simulink model "Buckfsattempt"  (R2022b)
settings: Solver=VariableStepAuto  StartTime=0.0  StopTime=2  RelTol=1e-3
values from neighbouring files (symbols this model uses):
  angular_corner_freq = ( (n^3*(1-D)^2*R_L + (n-D*(n-1)*r_l) ) / (L_m*C*(R_L + r_c)*(n-D*(n-1)) ) )^0.5    (= 137999.679282)    [Worspace.m]
  C_min = D/(R_L*fsw*Output_V_rip)    (= 9.6e-05)    [Worspace.m]
  D = 0.4    [Model_Worksapce.mat]    (also in Worspace.m = 0.5)
  damp_ratio = tau/(2*(rho*gamma)^0.5)    (= 0.148310872127)    [Worspace.m]
  fsw = 100000    [Model_Worksapce.mat]    (also in Worspace.m)
  Gain_Constant = ( (n^2*D*D_n*R_L*r_c ) / (L_m*(R_L + r_c)*(n-D*(n-1))) )    (= 22245.3945082)    [Worspace.m]
  L_m = 0.25    [Model_Worksapce.mat]    (also in Worspace.m = 3.41796875e-07)
  N1 = 24    [Model_Worksapce.mat]    (also in Worspace.m)
  N2 = 72    [Model_Worksapce.mat]    (also in Worspace.m = 48)
  N2_N1 = 3    [Model_Worksapce.mat]    (also in Worspace.m = 2)
  P_out = 50    [Model_Worksapce.mat]    (also in Worspace.m)
  R_L = 1.04166666667    [Model_Worksapce.mat]    (also in Worspace.m)
  Vs = 24    [Model_Worksapce.mat]    (also in Worspace.m)
  w_zn = 1/(C*r_c)    (= 104166.666667)    [Worspace.m]
libraries: spsCurrentMeasurementLib x10, spsSeriesRLCBranchLib x10, spsVoltageMeasurementLib x7, spsDCVoltageSourceLib x5, spsControlledCurrentSourceLib x2, spsControlledVoltageSourceLib x2, spsDiodeLib x2, spsIdealSwitchLib x2, spsMeanLib x2, spsPWMGeneratorDCDCLib x2, spsParallelRLCBranchLib x1, spsLinearTransformerLib x1
settings Model: Creator=enese  LastModifiedBy=enese

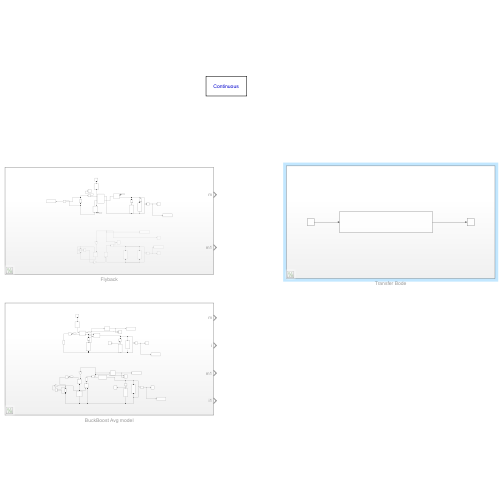
[thumbnail: Simulink's stored preview of the top-level diagram]
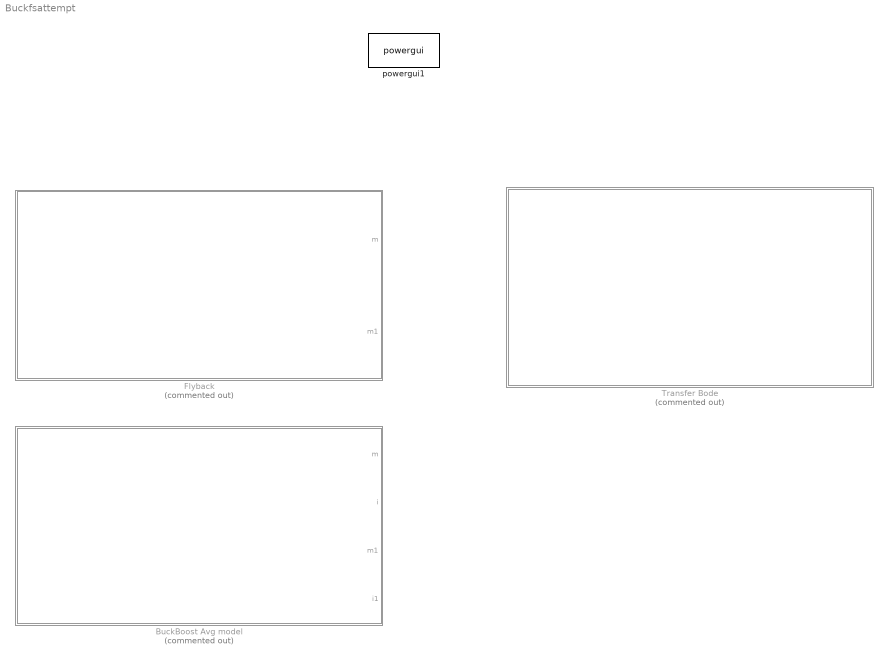
== system Buckfsattempt ==
  BuckBoost Avg model : Subsystem  Commented=on
  Flyback : Subsystem  Commented=on
  Transfer Bode : Subsystem  Commented=on
  powergui1 : spspowerguiLib/powergui  Priority=1  SimulationMode=Continuous  SampleTime=50e-6  frequency=60  Iterations=50  frequencyindice=0  Pbase=100e6  ErrMax=1e-4  UnitsV=kV  UnitsW=MW  buscounter=0  FunctionMessages=off  echomessages=off  EnableUseOfTLC=off  CurrentSourceSwitches=off  DisableSnubberDevices=off  DisableRonSwitches=off  DisableVfSwitches=off  DisplayEquations=off  AutomaticDiscreteSolvers=off  SolverType=Tustin/Backward Euler (TBE)  Interpol=off  ExternalGateDelay=off  methode=off  Ts=100  x0status=blocks  SPID=on  SwTol=0  HookPort=off  NonlinearTolerance=1e-4  nMaxIteration=100  ContinueOnMaxIteration=off  RestoreLinks=warning  ResistiveCurrentMeasurement=off  Frange=[0:2:500]  Ylog=off  Xlog=on  ShowGrid=off  save=off  variable=ZData  structure=0  ZoomFFT=off  StartTime=0.0  cycles=1  DisplayStyle=1  fundamental=60  FreqAxis=off  MaxFrequency=1000  frequencyindicesteady=1  RmsSteady=1  display=off

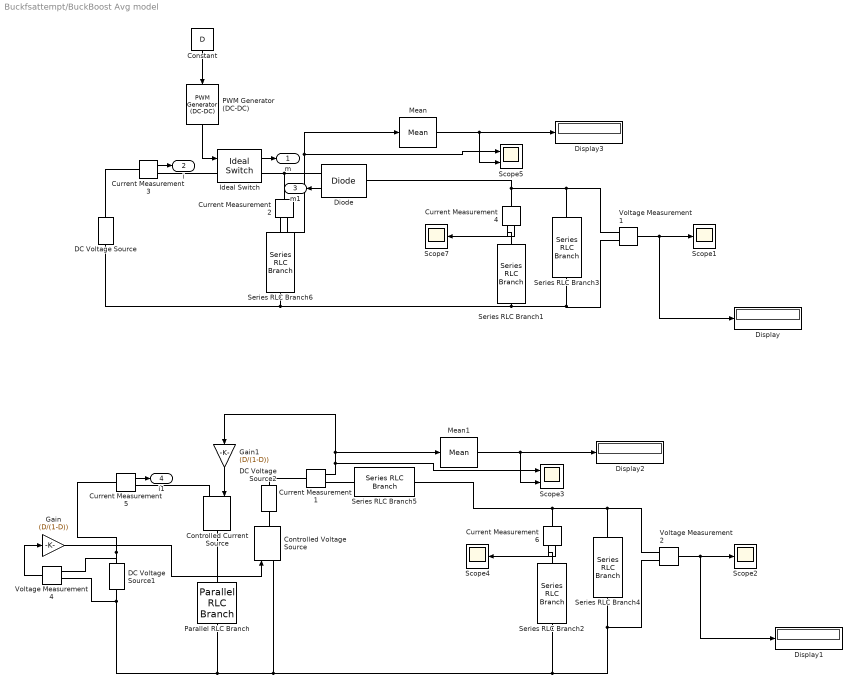
== system Buckfsattempt/BuckBoost Avg model ==
  Constant : Constant  Value=D
  Controlled Current Source : spsControlledCurrentSourceLib/Controlled Current Source  Initialize=on  Source_Type=DC  Amplitude=0  Phase=0  Frequency=0  Measurements=None
  Controlled Voltage Source : spsControlledVoltageSourceLib/Controlled Voltage Source  Initialize=on  Source_Type=DC  Amplitude=0  Phase=0  Frequency=0  Measurements=None
  Current Measurement{1..6} (6 alike) : spsCurrentMeasurementLib/Current Measurement  PhasorSimulation=off  OutputType=Complex  PSBequivalent=0
  DC Voltage Source : spsDCVoltageSourceLib/DC Voltage Source  Amplitude=Vs  Measurements=Voltage
  DC Voltage Source1 : spsDCVoltageSourceLib/DC Voltage Source  Amplitude=Vs  Measurements=Voltage
  DC Voltage Source2 : spsDCVoltageSourceLib/DC Voltage Source  Amplitude=0  Measurements=Voltage
  Diode : spsDiodeLib/Diode  Ron=0.001  Lon=0  Vf=0.8  IC=0  UseSnubber=0  Rs=500  Cs=250e-9  Measurements=on
  Display{,1..3} (4 alike) : Display
  Gain : Gain  Gain=(D/(1-D))
  Gain1 : Gain  Gain=(D/(1-D))
  Ideal Switch : spsIdealSwitchLib/Ideal Switch  Ron=0.001  Lon=0  IC=0  Rs=1e5  Cs=inf  Measurements=on
  Mean : spsMeanLib/Mean  Freq=100e3  Vinit=0  Ts=0
  Mean1 : spsMeanLib/Mean  Freq=100e3  Vinit=0  Ts=0
  PWM Generator (DC-DC) : spsPWMGeneratorDCDCLib/PWM Generator (DC-DC)  Fsw=100e3  Ts=0
  Parallel RLC Branch : spsParallelRLCBranchLib/Parallel RLC Branch  LConnTagsString=a  RConnTagsString=__new0  BranchType=RL  Resistance=1e10  Inductance=20e-6  SetiL0=off  InitialCurrent=0  Capacitance=1e-6  Setx0=off  InitialVoltage=0  Measurements=None
  Scope{1..2,4,7} (4 alike) : Scope
  Scope3 : Scope  NumInputPorts=2
  Scope5 : Scope  NumInputPorts=2
  Series RLC Branch1 : spsSeriesRLCBranchLib/Series RLC Branch  LConnTagsString=__new0  RConnTagsString=__new0  BranchType=C  Resistance=50e-7  Inductance=1e-3  SetiL0=off  InitialCurrent=0  Capacitance=80e-6  Setx0=off  InitialVoltage=0  Measurements=None
  Series RLC Branch2 : spsSeriesRLCBranchLib/Series RLC Branch  LConnTagsString=__new0  RConnTagsString=__new0  BranchType=C  Resistance=50e-7  Inductance=1e-3  SetiL0=off  InitialCurrent=0  Capacitance=80e-6  Setx0=off  InitialVoltage=0  Measurements=None
  Series RLC Branch3 : spsSeriesRLCBranchLib/Series RLC Branch  LConnTagsString=__new0  RConnTagsString=__new0  BranchType=R  Resistance=5  Inductance=1e-3  SetiL0=off  InitialCurrent=0  Capacitance=20e-6  Setx0=off  InitialVoltage=0  Measurements=None
  Series RLC Branch4 : spsSeriesRLCBranchLib/Series RLC Branch  LConnTagsString=__new0  RConnTagsString=__new0  BranchType=R  Resistance=5  Inductance=1e-3  SetiL0=off  InitialCurrent=0  Capacitance=20e-6  Setx0=off  InitialVoltage=0  Measurements=None
  Series RLC Branch5 : spsSeriesRLCBranchLib/Series RLC Branch  LConnTagsString=__new0  RConnTagsString=__new0  BranchType=L  Resistance=50e-7  Inductance=1e-3  SetiL0=off  InitialCurrent=0  Capacitance=80e-6  Setx0=off  InitialVoltage=0  Measurements=None
  Series RLC Branch6 : spsSeriesRLCBranchLib/Series RLC Branch  LConnTagsString=__new0  RConnTagsString=__new0  BranchType=L  Resistance=50e-7  Inductance=20e-6  SetiL0=off  InitialCurrent=0  Capacitance=470e-6  Setx0=off  InitialVoltage=0  Measurements=None
  Voltage Measurement1 : spsVoltageMeasurementLib/Voltage Measurement  PhasorSimulation=off  OutputType=Complex  PSBequivalent=0
  Voltage Measurement2 : spsVoltageMeasurementLib/Voltage Measurement  PhasorSimulation=off  OutputType=Complex  PSBequivalent=0
  Voltage Measurement4 : spsVoltageMeasurementLib/Voltage Measurement  PhasorSimulation=off  OutputType=Complex  PSBequivalent=0
  m : Outport
  i : Outport  Port=2
  m1 : Outport  Port=3
  i1 : Outport  Port=4
  wires:
  Gain/1 -> Controlled Voltage Source/1
  PWM Generator (DC-DC)/1 -> Ideal Switch/1
  Mean1/1 -> Display2/1, Scope3/2
  Voltage Measurement4/1 -> Gain/1
  Ideal Switch/1 -> m/1
  Voltage Measurement1/1 -> Scope1/1, Display/1
  Constant/1 -> PWM Generator (DC-DC)/1
  Current Measurement1/1 -> Scope3/1, Mean1/1, Gain1/1
  Voltage Measurement2/1 -> Display1/1, Scope2/1
  Gain1/1 -> Controlled Current Source/1
  Current Measurement4/1 -> Scope7/1
  Mean/1 -> Scope5/2, Display3/1
  Current Measurement2/1 -> Mean/1, Scope5/1
  Current Measurement6/1 -> Scope4/1
  Current Measurement3/1 -> i/1
  Diode/1 -> m1/1
  Current Measurement5/1 -> i1/1
  connections:
  Ideal Switch/RConn1 -- Current Measurement2/LConn1 -- Diode/RConn1
  Current Measurement6/RConn1 -- Series RLC Branch2/LConn1
  Voltage Measurement2/LConn2 -- Series RLC Branch4/RConn1 -- Series RLC Branch2/RConn1 -- Parallel RLC Branch/RConn1 -- Voltage Measurement4/LConn1 -- DC Voltage Source1/LConn1 -- Controlled Voltage Source/LConn1
  Voltage Measurement2/LConn1 -- Series RLC Branch4/LConn1 -- Series RLC Branch5/RConn1 -- Current Measurement6/LConn1
  Series RLC Branch3/RConn1 -- DC Voltage Source/LConn1 -- Series RLC Branch6/LConn1 -- Series RLC Branch1/RConn1 -- Voltage Measurement1/LConn2
  Current Measurement2/RConn1 -- Series RLC Branch6/RConn1
  Current Measurement1/LConn1 -- DC Voltage Source2/RConn1
  Series RLC Branch5/LConn1 -- Current Measurement1/RConn1
  Voltage Measurement1/LConn1 -- Diode/LConn1 -- Current Measurement4/LConn1 -- Series RLC Branch3/LConn1
  Current Measurement5/LConn1 -- Voltage Measurement4/LConn2 -- DC Voltage Source1/RConn1
  Current Measurement4/RConn1 -- Series RLC Branch1/LConn1
  Ideal Switch/LConn1 -- Current Measurement3/RConn1
  Controlled Current Source/LConn1 -- Current Measurement5/RConn1
  Current Measurement3/LConn1 -- DC Voltage Source/RConn1
  Parallel RLC Branch/LConn1 -- Controlled Current Source/RConn1
  DC Voltage Source2/LConn1 -- Controlled Voltage Source/RConn1

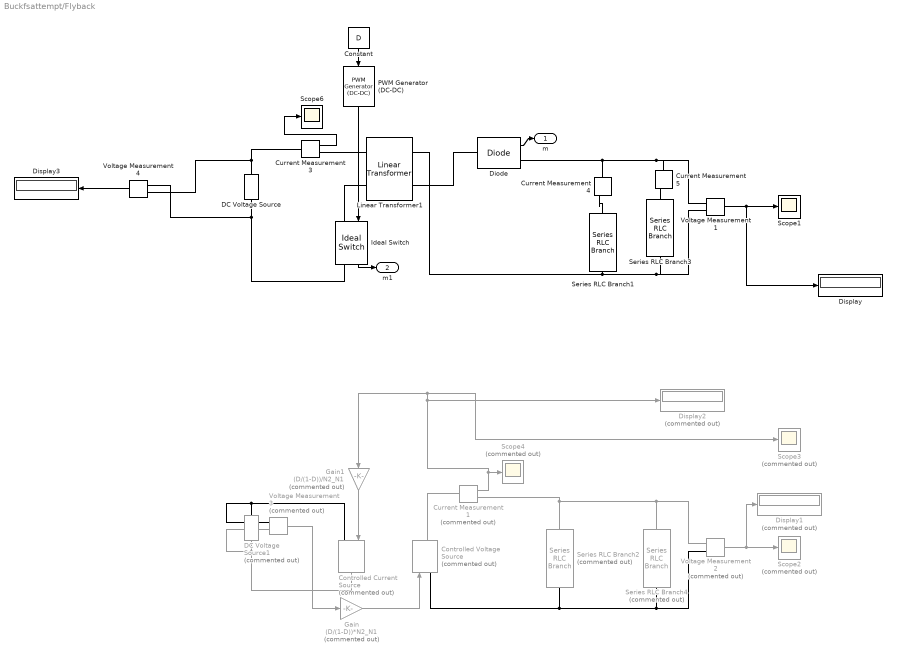
== system Buckfsattempt/Flyback ==
  Constant : Constant  Value=D
  Controlled Current Source : spsControlledCurrentSourceLib/Controlled Current Source  Commented=on  Initialize=on  Source_Type=DC  Amplitude=0  Phase=0  Frequency=0  Measurements=None
  Controlled Voltage Source : spsControlledVoltageSourceLib/Controlled Voltage Source  Commented=on  Initialize=on  Source_Type=DC  Amplitude=0  Phase=0  Frequency=0  Measurements=None
  Current Measurement1 : spsCurrentMeasurementLib/Current Measurement  Commented=on  PhasorSimulation=off  OutputType=Complex  PSBequivalent=0
  Current Measurement3 : spsCurrentMeasurementLib/Current Measurement  PhasorSimulation=off  OutputType=Complex  PSBequivalent=0
  Current Measurement4 : spsCurrentMeasurementLib/Current Measurement  PhasorSimulation=off  OutputType=Complex  PSBequivalent=0
  Current Measurement5 : spsCurrentMeasurementLib/Current Measurement  PhasorSimulation=off  OutputType=Complex  PSBequivalent=0
  DC Voltage Source : spsDCVoltageSourceLib/DC Voltage Source  Amplitude=Vs  Measurements=Voltage
  DC Voltage Source1 : spsDCVoltageSourceLib/DC Voltage Source  Commented=on  Amplitude=Vs  Measurements=Voltage
  Diode : spsDiodeLib/Diode  Ron=0.001  Lon=0  Vf=0.8  IC=0  UseSnubber=0  Rs=800  Cs=250e-9  Measurements=on
  Display : Display
  Display1 : Display  Commented=on
  Display2 : Display  Commented=on
  Display3 : Display
  Gain : Gain  Commented=on  Gain=(D/(1-D))*N2_N1
  Gain1 : Gain  Commented=on  Gain=(D/(1-D))/N2_N1
  Ideal Switch : spsIdealSwitchLib/Ideal Switch  Ron=0.001  Lon=0  IC=0  Rs=1e5  Cs=inf  Measurements=on
  Linear Transformer1 : spsLinearTransformerLib/Linear Transformer  UNITS=SI  NominalPower=[ P_out fsw ]  winding1=[N1 0 0]  winding2="[N2 0  0]"  ThreeWindings=off  winding3=[3.15e+05 3.969e+07 6316.9]  RmLm=[10e8 L_m*1.05]  Measurements=None  DataType=on
  PWM Generator (DC-DC) : spsPWMGeneratorDCDCLib/PWM Generator (DC-DC)  Fsw=fsw  Ts=0
  Scope1 : Scope
  Scope2 : Scope  Commented=on
  Scope3 : Scope  Commented=on
  Scope4 : Scope  Commented=on
  Scope6 : Scope
  Series RLC Branch1 : spsSeriesRLCBranchLib/Series RLC Branch  LConnTagsString=__new0  RConnTagsString=__new0  BranchType=RC  Resistance=50e-8  Inductance=1e-3  SetiL0=off  InitialCurrent=0  Capacitance=C_min  Setx0=off  InitialVoltage=0  Measurements=None
  Series RLC Branch2 : spsSeriesRLCBranchLib/Series RLC Branch  Commented=on  LConnTagsString=__new0  RConnTagsString=__new0  BranchType=RC  Resistance=50e-7  Inductance=1e-3  SetiL0=off  InitialCurrent=0  Capacitance=470e-6  Setx0=off  InitialVoltage=0  Measurements=None
  Series RLC Branch3 : spsSeriesRLCBranchLib/Series RLC Branch  LConnTagsString=__new0  RConnTagsString=__new0  BranchType=R  Resistance=R_L  Inductance=1e-3  SetiL0=off  InitialCurrent=0  Capacitance=20e-6  Setx0=off  InitialVoltage=0  Measurements=None
  Series RLC Branch4 : spsSeriesRLCBranchLib/Series RLC Branch  Commented=on  LConnTagsString=__new0  RConnTagsString=__new0  BranchType=R  Resistance=5  Inductance=1e-3  SetiL0=off  InitialCurrent=0  Capacitance=20e-6  Setx0=off  InitialVoltage=0  Measurements=None
  Voltage Measurement1 : spsVoltageMeasurementLib/Voltage Measurement  PhasorSimulation=off  OutputType=Complex  PSBequivalent=0
  Voltage Measurement2 : spsVoltageMeasurementLib/Voltage Measurement  Commented=on  PhasorSimulation=off  OutputType=Complex  PSBequivalent=0
  Voltage Measurement3 : spsVoltageMeasurementLib/Voltage Measurement  Commented=on  PhasorSimulation=off  OutputType=Complex  PSBequivalent=0
  Voltage Measurement4 : spsVoltageMeasurementLib/Voltage Measurement  PhasorSimulation=off  OutputType=Complex  PSBequivalent=0
  m : Outport
  m1 : Outport  Port=2
  wires:
  Current Measurement3/1 -> Scope6/1
  Current Measurement1/1 -> Display2/1, Scope3/1, Gain1/1, Scope4/1
  Gain/1 -> Controlled Voltage Source/1
  Voltage Measurement2/1 -> Display1/1, Scope2/1
  Diode/1 -> m/1
  Voltage Measurement3/1 -> Gain/1
  Voltage Measurement1/1 -> Display/1, Scope1/1
  Constant/1 -> PWM Generator (DC-DC)/1
  PWM Generator (DC-DC)/1 -> Ideal Switch/1
  Gain1/1 -> Controlled Current Source/1
  Ideal Switch/1 -> m1/1
  Voltage Measurement4/1 -> Display3/1
  connections:
  Current Measurement4/RConn1 -- Series RLC Branch1/LConn1
  Ideal Switch/RConn1 -- Voltage Measurement4/LConn2 -- DC Voltage Source/LConn1
  Current Measurement4/LConn1 -- Diode/RConn1 -- Voltage Measurement1/LConn1 -- Current Measurement5/LConn1
  Current Measurement3/RConn1 -- Linear Transformer1/LConn1
  DC Voltage Source1/RConn1 -- Controlled Current Source/LConn1 -- Voltage Measurement3/LConn1
  Series RLC Branch2/RConn1 -- Controlled Voltage Source/LConn1 -- Series RLC Branch4/RConn1 -- Voltage Measurement2/LConn2
  Voltage Measurement2/LConn1 -- Series RLC Branch4/LConn1 -- Current Measurement1/RConn1 -- Series RLC Branch2/LConn1
  Ideal Switch/LConn1 -- Linear Transformer1/LConn2
  Current Measurement1/LConn1 -- Controlled Voltage Source/RConn1
  Current Measurement3/LConn1 -- Voltage Measurement4/LConn1 -- DC Voltage Source/RConn1
  Linear Transformer1/RConn2 -- Diode/LConn1
  Linear Transformer1/RConn1 -- Series RLC Branch3/RConn1 -- Voltage Measurement1/LConn2 -- Series RLC Branch1/RConn1
  Voltage Measurement3/LConn2 -- Controlled Current Source/RConn1 -- DC Voltage Source1/LConn1
  Current Measurement5/RConn1 -- Series RLC Branch3/LConn1

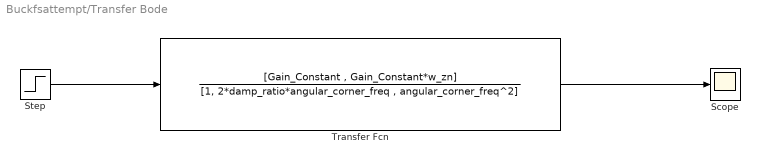
== system Buckfsattempt/Transfer Bode ==
  Scope : Scope
  Step : Step  SampleTime=0
  Transfer Fcn : TransferFcn  Numerator=[Gain_Constant , Gain_Constant*w_zn]  Denominator=[1, 2*damp_ratio*angular_corner_freq , angular_corner_freq^2]
  wires:
  Step/1 -> Transfer Fcn/1
  Transfer Fcn/1 -> Scope/1
